simulink model "EV_PowerFlowSystemArch"  (R2023a)
settings: configuration reference "Configuration" (kept outside this file)
settings Model: DataDictionary=ZC_EVPowerSystem.sldd  Creator=ykamatan  LastModifiedBy=ykamatan
settings ConfigSetRef: SourceName=Configuration

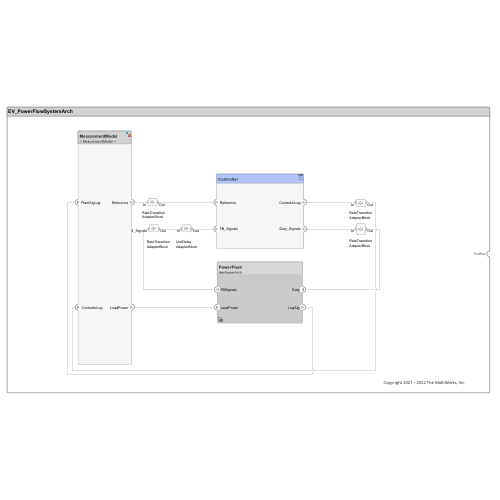
[thumbnail: Simulink's stored preview of the top-level diagram]
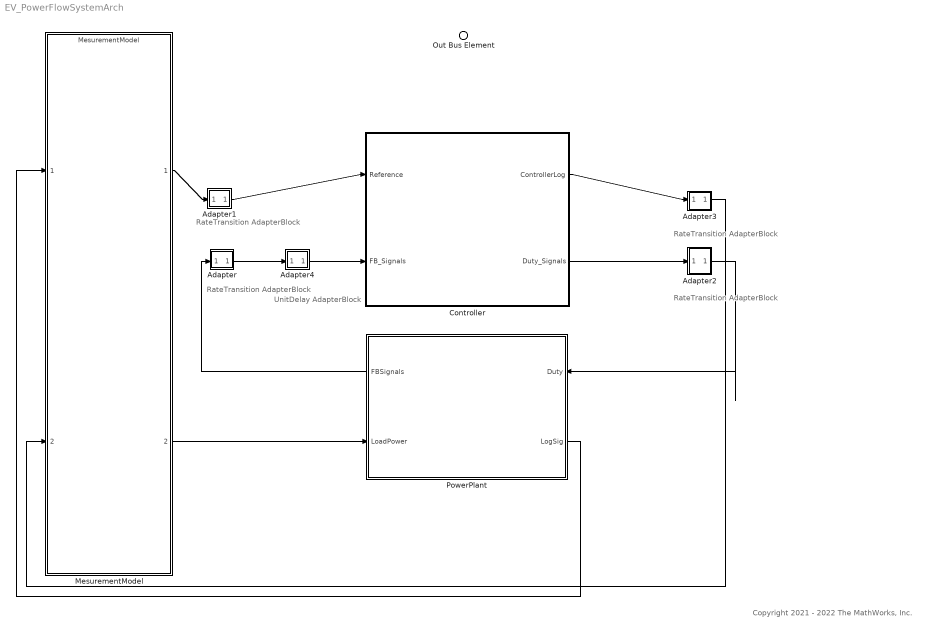
== system EV_PowerFlowSystemArch ==
  note: Copyright 2021 - 2022 The MathWorks, Inc.
  note: RateTransition
      | AdapterBlock
  note: RateTransition
      | AdapterBlock
  note: RateTransition
      | AdapterBlock
  note: RateTransition
      | AdapterBlock
  note: UnitDelay
      | AdapterBlock
  Adapter : Subsystem
      settings: PortSchema="{\"entries\":[{\"content\":{\"margin\":10,\"minimumSpacing\":15,\"sides\":[{\"content\":{\"connectorIds\":[\"In1\"]},\"type\":\"ConnectorPlacement.EquallySpacedRectSide\",\"uuid\":\"83593e86-a1ca-46ab-bb48-ac1b1e7f94a6\"},{\"content\":{\"connectorIds\":[\"Out1\"],\"side\":\"RIGHT\"},\"type\":\"ConnectorPlacement.EquallySpacedRectSide\",\"uuid\":\"814b1f5e-b094-459d-8c9a-0a4f126f7c52\"},{\"content\":{\"connectorIds\":[],\"side\":\"TOP\"},\"type\":\"ConnectorPlacement.EquallySpacedRectSide\",\"uuid\":\"69a5ca39-2f24-4b9e-8cab-6a5451834002\"}]},\"type\":\"ConnectorPlacement.EquallySpacedConnector\",\"uuid\":\"00154813-bb7b-4bb4-a499-13c3b926de90\"}],\"packageUris\":[\"http://schema.mathworks.com/mf0/Connector/R2020b\"],\"version\":\"1.0\"}"
  Adapter1 : Subsystem
      settings: PortSchema="{\"entries\":[{\"content\":{\"margin\":10,\"minimumSpacing\":15,\"sides\":[{\"content\":{\"connectorIds\":[\"In1\"]},\"type\":\"ConnectorPlacement.EquallySpacedRectSide\",\"uuid\":\"47e0bb57-e194-4de3-af35-f87a70f6b467\"},{\"content\":{\"connectorIds\":[\"Out1\"],\"side\":\"RIGHT\"},\"type\":\"ConnectorPlacement.EquallySpacedRectSide\",\"uuid\":\"c2f19e85-f0e5-4ac0-8689-0748833037f0\"},{\"content\":{\"connectorIds\":[],\"side\":\"TOP\"},\"type\":\"ConnectorPlacement.EquallySpacedRectSide\",\"uuid\":\"48f24ce0-262a-4b1f-8d65-bd4861d2ae99\"}]},\"type\":\"ConnectorPlacement.EquallySpacedConnector\",\"uuid\":\"f77ce64d-7cae-42e1-8a92-44d91f0f1633\"}],\"packageUris\":[\"http://schema.mathworks.com/mf0/Connector/R2020b\"],\"version\":\"1.0\"}"
  Adapter2 : Subsystem
      settings: PortSchema="{\"entries\":[{\"content\":{\"margin\":10,\"minimumSpacing\":15,\"sides\":[{\"content\":{\"connectorIds\":[\"In1\"]},\"type\":\"ConnectorPlacement.EquallySpacedRectSide\",\"uuid\":\"38efb45f-a9c4-4617-9d8c-27c4cd9f3f1d\"},{\"content\":{\"connectorIds\":[\"Out1\"],\"side\":\"RIGHT\"},\"type\":\"ConnectorPlacement.EquallySpacedRectSide\",\"uuid\":\"11f6e9d9-e3f2-4ac6-90a7-b7d8cdb9c6c6\"},{\"content\":{\"connectorIds\":[],\"side\":\"TOP\"},\"type\":\"ConnectorPlacement.EquallySpacedRectSide\",\"uuid\":\"c47f34dd-9c13-4f03-82ea-3d6dfa7a9b5d\"}]},\"type\":\"ConnectorPlacement.EquallySpacedConnector\",\"uuid\":\"cdc19c7f-2efd-4227-b9c6-7a8f68375178\"}],\"packageUris\":[\"http://schema.mathworks.com/mf0/Connector/R2020b\"],\"version\":\"1.0\"}"
  Adapter3 : Subsystem
      settings: PortSchema="{\"entries\":[{\"content\":{\"margin\":10,\"minimumSpacing\":15,\"sides\":[{\"content\":{\"connectorIds\":[\"In1\"]},\"type\":\"ConnectorPlacement.EquallySpacedRectSide\",\"uuid\":\"47e0bb57-e194-4de3-af35-f87a70f6b467\"},{\"content\":{\"connectorIds\":[\"Out1\"],\"side\":\"RIGHT\"},\"type\":\"ConnectorPlacement.EquallySpacedRectSide\",\"uuid\":\"c2f19e85-f0e5-4ac0-8689-0748833037f0\"},{\"content\":{\"connectorIds\":[],\"side\":\"TOP\"},\"type\":\"ConnectorPlacement.EquallySpacedRectSide\",\"uuid\":\"48f24ce0-262a-4b1f-8d65-bd4861d2ae99\"}]},\"type\":\"ConnectorPlacement.EquallySpacedConnector\",\"uuid\":\"f77ce64d-7cae-42e1-8a92-44d91f0f1633\"}],\"packageUris\":[\"http://schema.mathworks.com/mf0/Connector/R2020b\"],\"version\":\"1.0\"}"
  Adapter4 : Subsystem
      settings: PortSchema="{\"entries\":[{\"content\":{\"margin\":10,\"minimumSpacing\":15,\"sides\":[{\"content\":{\"connectorIds\":[\"In1\"]},\"type\":\"ConnectorPlacement.EquallySpacedRectSide\",\"uuid\":\"47e0bb57-e194-4de3-af35-f87a70f6b467\"},{\"content\":{\"connectorIds\":[\"Out1\"],\"side\":\"RIGHT\"},\"type\":\"ConnectorPlacement.EquallySpacedRectSide\",\"uuid\":\"c2f19e85-f0e5-4ac0-8689-0748833037f0\"},{\"content\":{\"connectorIds\":[],\"side\":\"TOP\"},\"type\":\"ConnectorPlacement.EquallySpacedRectSide\",\"uuid\":\"48f24ce0-262a-4b1f-8d65-bd4861d2ae99\"}]},\"type\":\"ConnectorPlacement.EquallySpacedConnector\",\"uuid\":\"f77ce64d-7cae-42e1-8a92-44d91f0f1633\"}],\"packageUris\":[\"http://schema.mathworks.com/mf0/Connector/R2020b\"],\"version\":\"1.0\"}"
  Controller : Subsystem
      settings: PortSchema="{\"entries\":[{\"content\":{\"headerSize\":26,\"margin\":15,\"minimumSpacing\":25,\"sides\":[{\"content\":{\"connectorIds\":[\"In1\",\"In2\"]},\"type\":\"ConnectorPlacement.EquallySpacedRectSide\",\"uuid\":\"83593e86-a1ca-46ab-bb48-ac1b1e7f94a6\"},{\"content\":{\"connectorIds\":[\"Out1\",\"Out2\"],\"side\":\"RIGHT\"},\"type\":\"ConnectorPlacement.EquallySpacedRectSide\",\"uuid\":\"814b1f5e-b094-459d-8c9a-0a4f126f7c52\"},{\"content\":{\"connectorIds\":[],\"side\":\"TOP\"},\"type\":\"ConnectorPlacement.EquallySpacedRectSide\",\"uuid\":\"69a5ca39-2f24-4b9e-8cab-6a5451834002\"}]},\"type\":\"ConnectorPlacement.EquallySpacedConnector\",\"uuid\":\"00154813-bb7b-4bb4-a499-13c3b926de90\"}],\"packageUris\":[\"http://schema.mathworks.com/mf0/Connector/R2020b\"],\"version\":\"1.0\"}"
  MesurementModel : ModelReference  ModelNameDialog=MesurementModel  SimulationMode=Normal  ModelReferenceVersion=5.0
      settings: PortSchema="{\"entries\":[{\"content\":{\"headerSize\":38,\"margin\":15,\"minimumSpacing\":25,\"sides\":[{\"content\":{\"connectorIds\":[\"In1\",\"In2\"]},\"type\":\"ConnectorPlacement.EquallySpacedRectSide\",\"uuid\":\"38efb45f-a9c4-4617-9d8c-27c4cd9f3f1d\"},{\"content\":{\"connectorIds\":[\"Out1\",\"Out2\"],\"side\":\"RIGHT\"},\"type\":\"ConnectorPlacement.EquallySpacedRectSide\",\"uuid\":\"11f6e9d9-e3f2-4ac6-90a7-b7d8cdb9c6c6\"},{\"content\":{\"connectorIds\":[],\"side\":\"TOP\"},\"type\":\"ConnectorPlacement.EquallySpacedRectSide\",\"uuid\":\"c47f34dd-9c13-4f03-82ea-3d6dfa7a9b5d\"}]},\"type\":\"ConnectorPlacement.EquallySpacedConnector\",\"uuid\":\"cdc19c7f-2efd-4227-b9c6-7a8f68375178\"}],\"packageUris\":[\"http://schema.mathworks.com/mf0/Connector/R2020b\"],\"version\":\"1.0\"}"
  PowerPlant : Subsystem  Variant=on  VariantControlMode=label  VariantControl=Choice  LabelModeActiveChoice=HardwareArch
      settings: PortSchema="{\"entries\":[{\"content\":{\"headerSize\":38,\"margin\":15,\"minimumSpacing\":25,\"sides\":[{\"content\":{\"connectorIds\":[\"Out1\",\"In2\"]},\"type\":\"ConnectorPlacement.EquallySpacedRectSide\",\"uuid\":\"83593e86-a1ca-46ab-bb48-ac1b1e7f94a6\"},{\"content\":{\"connectorIds\":[\"In1\",\"Out2\"],\"side\":\"RIGHT\"},\"type\":\"ConnectorPlacement.EquallySpacedRectSide\",\"uuid\":\"814b1f5e-b094-459d-8c9a-0a4f126f7c52\"},{\"content\":{\"connectorIds\":[],\"side\":\"TOP\"},\"type\":\"ConnectorPlacement.EquallySpacedRectSide\",\"uuid\":\"69a5ca39-2f24-4b9e-8cab-6a5451834002\"}]},\"type\":\"ConnectorPlacement.EquallySpacedConnector\",\"uuid\":\"00154813-bb7b-4bb4-a499-13c3b926de90\"}],\"packageUris\":[\"http://schema.mathworks.com/mf0/Connector/R2020b\"],\"version\":\"1.0\"}"
  Out Bus Element : Outport  PortName=OutBus
  wires:
  Controller/2(Duty_Signals) -> Adapter2/1(In)
  Adapter1/1(Out) -> Controller/1(Reference)
  MesurementModel/1 -> Adapter1/1(In)
  Controller/1(ControllerLog) -> Adapter3/1(In)
  Adapter4/1(Out) -> Controller/2(FB_Signals)
  Adapter/1(Out) -> Adapter4/1(In)
  Adapter2/1(Out) -> PowerPlant/1(Duty)
  MesurementModel/2 -> PowerPlant/2(LoadPower)
  PowerPlant/1(FBSignals) -> Adapter/1(FB_Signals)
  PowerPlant/2(LogSig) -> MesurementModel/1
  Adapter3/1(Out) -> MesurementModel/2

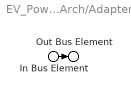
== system EV_PowerFlowSystemArch/Adapter ==
  In Bus Element : Inport  PortName=FB_Signals
  Out Bus Element : Outport  PortName=Out
  wires:
  In Bus Element/1 -> Out Bus Element/1

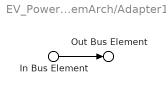
== system EV_PowerFlowSystemArch/Adapter1 ==
  In Bus Element : Inport  PortName=In
  Out Bus Element : Outport  PortName=Out
  wires:
  In Bus Element/1 -> Out Bus Element/1

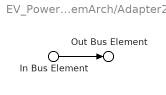
== system EV_PowerFlowSystemArch/Adapter2 ==
  In Bus Element : Inport  PortName=In
  Out Bus Element : Outport  PortName=Out
  wires:
  In Bus Element/1 -> Out Bus Element/1

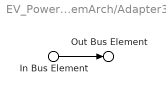
== system EV_PowerFlowSystemArch/Adapter3 ==
  In Bus Element : Inport  PortName=In
  Out Bus Element : Outport  PortName=Out
  wires:
  In Bus Element/1 -> Out Bus Element/1

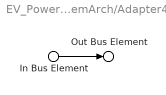
== system EV_PowerFlowSystemArch/Adapter4 ==
  In Bus Element : Inport  PortName=In
  Out Bus Element : Outport  PortName=Out
  wires:
  In Bus Element/1 -> Out Bus Element/1

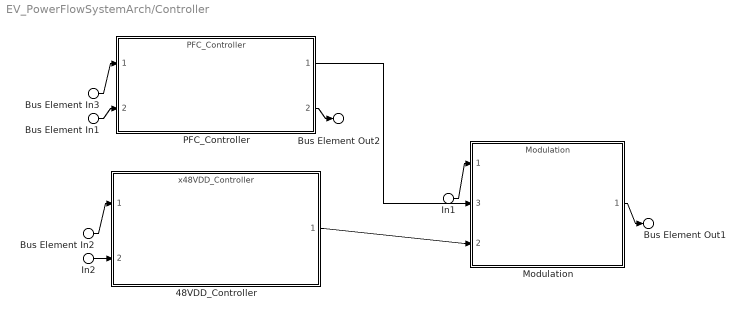
== system EV_PowerFlowSystemArch/Controller ==
  Bus Element In3 : Inport  PortName=Reference
  Bus Element In2 : Inport  PortName=Reference
  In1 : Inport  Port=2  PortName=FB_Signals
  In2 : Inport  Port=2  PortName=FB_Signals  Element=DD_FBSig
  Bus Element In1 : Inport  Port=2  PortName=FB_Signals  Element=PFC_FBSig
  48VDD_Controller : ModelReference  ModelNameDialog=x48VDD_Controller  SimulationMode=Normal  ModelReferenceVersion=5.0
      settings: PortSchema="{\"entries\":[{\"content\":{\"headerSize\":38,\"margin\":15,\"minimumSpacing\":25,\"sides\":[{\"content\":{\"connectorIds\":[\"In1\",\"In2\"]},\"type\":\"ConnectorPlacement.EquallySpacedRectSide\",\"uuid\":\"effce3b8-0d7f-4aa0-bb06-1db3c7ad72cd\"},{\"content\":{\"connectorIds\":[\"Out1\"],\"side\":\"RIGHT\"},\"type\":\"ConnectorPlacement.EquallySpacedRectSide\",\"uuid\":\"ff214e04-7c02-4f40-865f-6eb832682be6\"},{\"content\":{\"connectorIds\":[],\"side\":\"TOP\"},\"type\":\"ConnectorPlacement.EquallySpacedRectSide\",\"uuid\":\"bd06f79f-8baa-46d4-b537-777d1292c6d1\"}]},\"type\":\"ConnectorPlacement.EquallySpacedConnector\",\"uuid\":\"f86a5a3d-f244-458b-bed7-6fc0771dcc65\"}],\"packageUris\":[\"http://schema.mathworks.com/mf0/Connector/R2020b\"],\"version\":\"1.0\"}"
  Modulation : ModelReference  ModelNameDialog=Modulation  SimulationMode=Normal  ModelReferenceVersion=5.0
      settings: PortSchema="{\"entries\":[{\"content\":{\"headerSize\":38,\"margin\":15,\"minimumSpacing\":25,\"sides\":[{\"content\":{\"connectorIds\":[\"In1\",\"In3\",\"In2\"]},\"type\":\"ConnectorPlacement.EquallySpacedRectSide\",\"uuid\":\"38efb45f-a9c4-4617-9d8c-27c4cd9f3f1d\"},{\"content\":{\"connectorIds\":[\"Out1\"],\"side\":\"RIGHT\"},\"type\":\"ConnectorPlacement.EquallySpacedRectSide\",\"uuid\":\"11f6e9d9-e3f2-4ac6-90a7-b7d8cdb9c6c6\"},{\"content\":{\"connectorIds\":[],\"side\":\"TOP\"},\"type\":\"ConnectorPlacement.EquallySpacedRectSide\",\"uuid\":\"c47f34dd-9c13-4f03-82ea-3d6dfa7a9b5d\"}]},\"type\":\"ConnectorPlacement.EquallySpacedConnector\",\"uuid\":\"cdc19c7f-2efd-4227-b9c6-7a8f68375178\"}],\"packageUris\":[\"http://schema.mathworks.com/mf0/Connector/R2020b\"],\"version\":\"1.0\"}"
  PFC_Controller : ModelReference  ModelNameDialog=PFC_Controller  SimulationMode=Normal  ModelReferenceVersion=5.0
      settings: PortSchema="{\"entries\":[{\"content\":{\"headerSize\":38,\"margin\":15,\"minimumSpacing\":25,\"sides\":[{\"content\":{\"connectorIds\":[\"In1\",\"In2\"]},\"type\":\"ConnectorPlacement.EquallySpacedRectSide\",\"uuid\":\"effce3b8-0d7f-4aa0-bb06-1db3c7ad72cd\"},{\"content\":{\"connectorIds\":[\"Out1\",\"Out2\"],\"side\":\"RIGHT\"},\"type\":\"ConnectorPlacement.EquallySpacedRectSide\",\"uuid\":\"ff214e04-7c02-4f40-865f-6eb832682be6\"},{\"content\":{\"connectorIds\":[],\"side\":\"TOP\"},\"type\":\"ConnectorPlacement.EquallySpacedRectSide\",\"uuid\":\"bd06f79f-8baa-46d4-b537-777d1292c6d1\"}]},\"type\":\"ConnectorPlacement.EquallySpacedConnector\",\"uuid\":\"f86a5a3d-f244-458b-bed7-6fc0771dcc65\"}],\"packageUris\":[\"http://schema.mathworks.com/mf0/Connector/R2020b\"],\"version\":\"1.0\"}"
  Bus Element Out2 : Outport  PortName=ControllerLog
  Bus Element Out1 : Outport  Port=2  PortName=Duty_Signals
  wires:
  Bus Element In1/1 -> PFC_Controller/2
  Bus Element In3/1 -> PFC_Controller/1
  In2/1 -> 48VDD_Controller/2
  Bus Element In2/1 -> 48VDD_Controller/1
  48VDD_Controller/1 -> Modulation/2
  PFC_Controller/1 -> Modulation/3
  In1/1 -> Modulation/1
  Modulation/1 -> Bus Element Out1/1
  PFC_Controller/2 -> Bus Element Out2/1

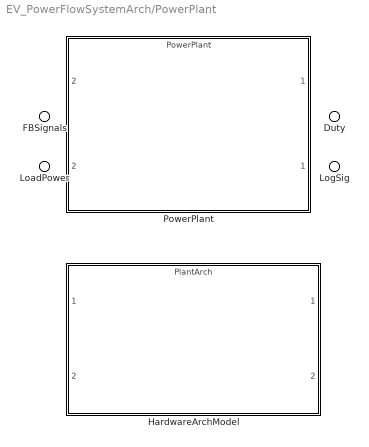
== system EV_PowerFlowSystemArch/PowerPlant ==
  Duty : Inport
  LoadPower : Inport  Port=2
  HardwareArchModel : ModelReference  ModelNameDialog=PlantArch  SimulationMode=Normal  VariantControl=HardwareArch  ModelReferenceVersion=4.0
      settings: PortSchema="{\"entries\":[{\"content\":{\"headerSize\":38,\"margin\":15,\"minimumSpacing\":25,\"sides\":[{\"content\":{\"connectorIds\":[\"In1\",\"In2\"]},\"type\":\"ConnectorPlacement.EquallySpacedRectSide\",\"uuid\":\"d44c4823-d533-41b7-9bc3-fb81246a6aac\"},{\"content\":{\"connectorIds\":[\"Out1\",\"Out2\"],\"side\":\"RIGHT\"},\"type\":\"ConnectorPlacement.EquallySpacedRectSide\",\"uuid\":\"f89a5651-3695-408a-bc6f-41b580c38d88\"},{\"content\":{\"connectorIds\":[],\"side\":\"TOP\"},\"type\":\"ConnectorPlacement.EquallySpacedRectSide\",\"uuid\":\"e8c09a01-263b-45e3-9851-fffab799fc47\"}]},\"type\":\"ConnectorPlacement.EquallySpacedConnector\",\"uuid\":\"675cb265-e806-4809-812b-3abe8e7f5533\"}],\"packageUris\":[\"http://schema.mathworks.com/mf0/Connector/R2020b\"],\"version\":\"1.0\"}"
  PowerPlant : ModelReference  ModelNameDialog=PowerPlant  SimulationMode=Normal  VariantControl=1DModel  ModelReferenceVersion=5.0
      settings: PortSchema="{\"entries\":[{\"content\":{\"headerSize\":38,\"margin\":15,\"minimumSpacing\":25,\"sides\":[{\"content\":{\"connectorIds\":[\"Out2\",\"In2\"]},\"type\":\"ConnectorPlacement.EquallySpacedRectSide\",\"uuid\":\"83593e86-a1ca-46ab-bb48-ac1b1e7f94a6\"},{\"content\":{\"connectorIds\":[\"In1\",\"Out1\"],\"side\":\"RIGHT\"},\"type\":\"ConnectorPlacement.EquallySpacedRectSide\",\"uuid\":\"814b1f5e-b094-459d-8c9a-0a4f126f7c52\"},{\"content\":{\"connectorIds\":[],\"side\":\"TOP\"},\"type\":\"ConnectorPlacement.EquallySpacedRectSide\",\"uuid\":\"69a5ca39-2f24-4b9e-8cab-6a5451834002\"}]},\"type\":\"ConnectorPlacement.EquallySpacedConnector\",\"uuid\":\"00154813-bb7b-4bb4-a499-13c3b926de90\"}],\"packageUris\":[\"http://schema.mathworks.com/mf0/Connector/R2020b\"],\"version\":\"1.0\"}"
  FBSignals : Outport
  LogSig : Outport  Port=2  OutDataTypeStr=Bus: PlantSigLog
